simulink model "project_7"  (R2020a)
settings: Solver=VariableStepAuto  StartTime=0.0  StopTime=Sim_Time  MaxStep=0.01  RelTol=1e-3
values from neighbouring files (symbols this model uses):
  b = 3.5077E-6    (= 3.5077e-06)    [project_10m.m]    (also in project_3m.m = 10; project_7m.m = 10; project_8m.m = 10; project_9m.m = 50)
  k = 20    [project_3m.m]    (also in project_7m.m; project_8m.m)
  Kd = 50    [project_7m.m]    (also in project_8m.m = 207.6; project_9m.m = 2)
  Ki = 300    [project_7m.m]    (also in project_8m.m = 7398; project_9m.m = 4)
  Kp = 1    [project_6m.m]    (also in project_7m.m = 350; project_8m.m = 4433; project_9m.m = 8000)
  m = 1    [project_3m.m]    (also in project_7m.m; project_8m.m; project_9m.m = 1000)
settings Model: Creator=Matt  LastModifiedBy=Matt
settings SolverCC: MaxConsecutiveMinStep=100
settings DataIOCC: ReturnWorkspaceOutputs=off  TimeSaveName=time

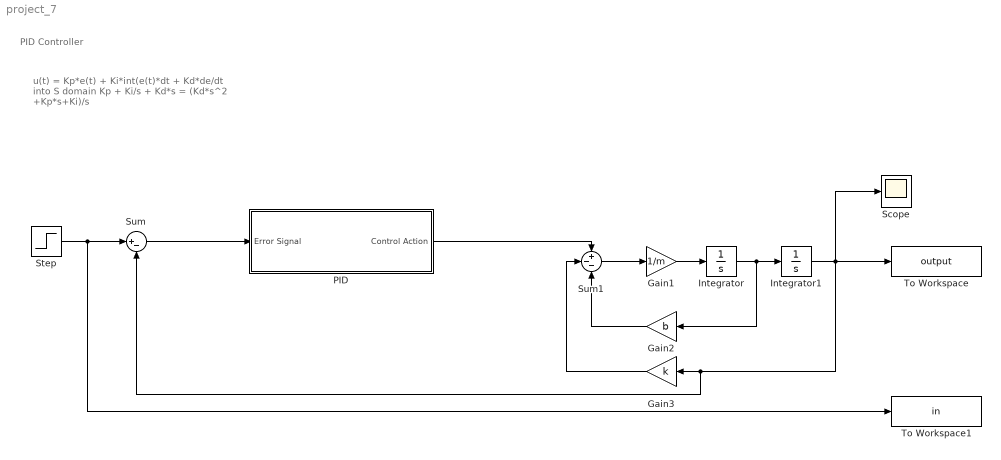
== system project_7 ==
  note: u(t) = Kp*e(t) + Ki*int(e(t)*dt + Kd*de/dt
      | into S domain
      | Kp + Ki/s + Kd*s = (Kd*s^2 +Kp*s+Ki)/s
  note: PID Controller
  Gain1 : Gain  Gain=1/m
  Gain2 : Gain  Gain=b
  Gain3 : Gain  Gain=k
  Integrator : Integrator
  Integrator1 : Integrator
  PID : Subsystem
  Scope : Scope
  Step : Step  SampleTime=0
  Sum : Sum  Inputs=|+-
  Sum1 : Sum  Inputs=+--
  To Workspace : ToWorkspace  VariableName=output  SampleTime=-1
  To Workspace1 : ToWorkspace  VariableName=in  SampleTime=-1
  wires:
  Sum/1 -> PID/1(Error Signal)
  PID/1(Control Action) -> Sum1/1
  Step/1 -> To Workspace1/1, Sum/1
  Sum1/1 -> Gain1/1
  Gain2/1 -> Sum1/3
  Gain3/1 -> Sum1/2
  Gain1/1 -> Integrator/1
  Integrator/1 -> Gain2/1, Integrator1/1
  Integrator1/1 -> Scope/1, To Workspace/1, Sum/2, Gain3/1

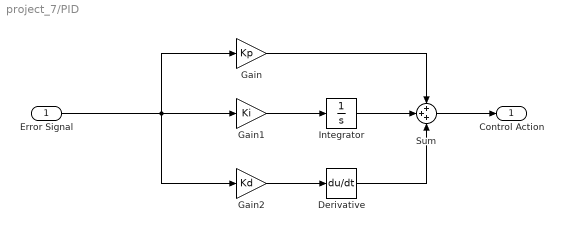
== system project_7/PID ==
  Error Signal : Inport
  Derivative : Derivative
  Gain : Gain  Gain=Kp
  Gain1 : Gain  Gain=Ki
  Gain2 : Gain  Gain=Kd
  Integrator : Integrator
  Sum : Sum  Inputs=+++
  Control Action : Outport
  wires:
  Derivative/1 -> Sum/3
  Error Signal/1 -> Gain2/1, Gain/1, Gain1/1
  Gain/1 -> Sum/1
  Sum/1 -> Control Action/1
  Integrator/1 -> Sum/2
  Gain1/1 -> Integrator/1
  Gain2/1 -> Derivative/1
